simulink model "Pt_Center_Diff_CS9"  (Simulink 7.6)
settings: Solver=ode45  StartTime=0  StopTime=20  FixedStep=TSTEP  RelTol=1e-3
PreLoadFcn:
  | cd Extensions/Simulink/pt_center_diff
  | Run_ft4wd_eclass
  | lsd_parameta_eclass
  | cd ../../..
undefined symbols (not defined in the file): LOCKED_XC_DAMP, LOCKED_XC_K, LOCKED_XC_OPT, M_DIFF_XC_TABLE, R_EFF_F_XC, R_EFF_R_XC, R_GEAR_XC, R_REAR_XC
libraries: Solver_SF x1
settings Model: Creator=ywata  LastModifiedBy=hkawanishi  ExtModeTrigMode=oneshot  ExtModeArmWhenConnect=off
settings DataIOCC: LimitDataPoints=off  SaveOutput=off  SaveTime=off  SignalLoggingName=sigsOut
settings OptimizationCC: BooleanDataType=off
settings DebuggingCC: SaveWithParameterizedLinksMsg=none  SignalResolutionControl=TryResolveAllWithWarning  SolverPrmCheckMsg=none  MultiTaskDSMMsg=warning  MultiTaskCondExecSysMsg=none  FcnCallInpInsideContextMsg=Enable All
settings HardwareCC: TargetUnknown=on
settings CodeAppCC: CustomSymbolStrType=$N$R$M_T
settings GRTTargetCC: TargetFcnLib=ansi_tfl_tmw.mat  TargetFunctionLibrary=C89/C90 (ANSI)  ModelReferenceCompliant=off  MatFileLogging=off

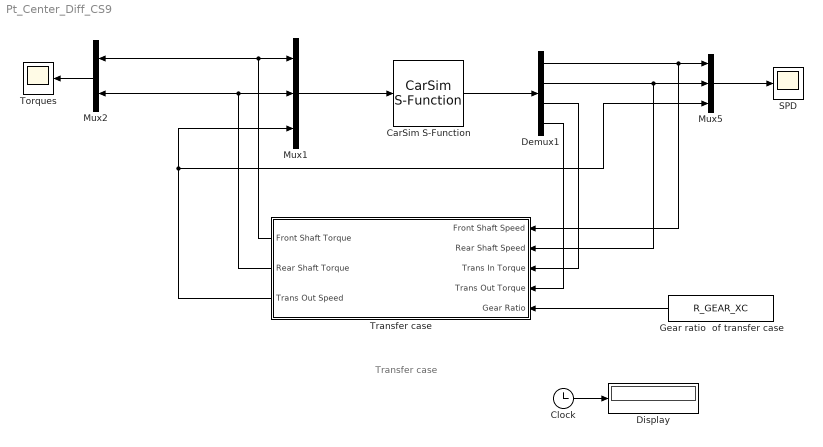
== system Pt_Center_Diff_CS9 ==
  note: Transfer case
  CarSim S-Function : Solver_SF/CarSim S-Function  Priority=1  SIMFILE=simfile.sim
  Clock : Clock
      settings: Decimation=10
  Demux1 : Demux
  Display : Display
  Gear ratio  of transfer case : Constant  Value=R_GEAR_XC
  Mux1 : Mux  Inputs=3
  Mux2 : Mux  Inputs=2
  Mux5 : Mux  Inputs=3
  SPD : Scope
      settings: YMin=-130.178  YMax=3627.22
  Torques : Scope
      settings: YMin=0  YMax=1200
  Transfer case : Subsystem
  wires:
  Mux2/1 -> Torques/1
  Mux5/1 -> SPD/1
  Gear ratio  of transfer case/1 -> Transfer case/5(Gear Ratio)
  Transfer case/3(Trans Out Speed) -> Mux1/3, Mux5/3
  Clock/1 -> Display/1
  CarSim S-Function/1 -> Demux1/1
  Mux1/1 -> CarSim S-Function/1
  Transfer case/1(Front Shaft Torque) -> Mux1/1, Mux2/1
  Transfer case/2(Rear Shaft Torque) -> Mux1/2, Mux2/2
  Demux1/1 -> Mux5/1, Transfer case/1(Front Shaft Speed)
  Demux1/2 -> Mux5/2, Transfer case/2(Rear Shaft Speed)
  Demux1/3 -> Transfer case/3(Trans In Torque)
  Demux1/4 -> Transfer case/4(Trans Out Torque)

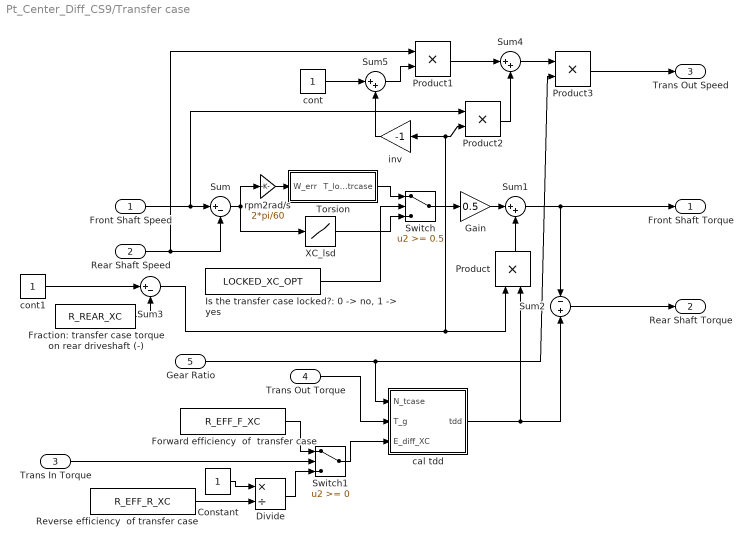
== system Pt_Center_Diff_CS9/Transfer case ==
  Front Shaft Speed : Inport
  Rear Shaft Speed : Inport  Port=2
  Trans In Torque : Inport  Port=3
  Trans Out Torque : Inport  Port=4
  Gear Ratio : Inport  Port=5
  Constant : Constant
  Divide : Product  Inputs=*/  InputSameDT=on  OutDataTypeStr=Inherit: Same as first input
  Forward efficiency  of  transfer case : Constant  Value=R_EFF_F_XC
  Fraction: transfer case torque on rear driveshaft (-) : Constant  Value=R_REAR_XC
  Gain : Gain  Gain=0.5  SaturateOnIntegerOverflow=on  OutDataTypeStr=Inherit: Same as input  ParamDataTypeStr=Inherit: Same as input
  "Is the transfer case locked?: 0 -> no, 1 -> yes" : Constant  Value=LOCKED_XC_OPT
  Product{,1..3} (4 alike) : Product  SaturateOnIntegerOverflow=on  InputSameDT=on  OutDataTypeStr=Inherit: Same as first input
  Reverse efficiency  of transfer case : Constant  Value=R_EFF_R_XC
  Sum : Sum  Inputs=|+-  SaturateOnIntegerOverflow=on  InputSameDT=on  OutDataTypeStr=Inherit: Same as first input
  Sum1 : Sum  Inputs=|++  SaturateOnIntegerOverflow=on  InputSameDT=on  OutDataTypeStr=Inherit: Same as first input
  Sum2 : Sum  Inputs=-|+  SaturateOnIntegerOverflow=on  InputSameDT=on  OutDataTypeStr=Inherit: Same as first input
  Sum3 : Sum  Inputs=|+-  SaturateOnIntegerOverflow=on  InputSameDT=on  OutDataTypeStr=Inherit: Same as first input
  Sum4 : Sum  Inputs=|++  SaturateOnIntegerOverflow=on  InputSameDT=on  OutDataTypeStr=Inherit: Same as first input
  Sum5 : Sum  Inputs=|++  SaturateOnIntegerOverflow=on  InputSameDT=on  OutDataTypeStr=Inherit: Same as first input
  Switch : Switch  Threshold=0.5  SaturateOnIntegerOverflow=on  InputSameDT=on
  Switch1 : Switch  SaturateOnIntegerOverflow=on  InputSameDT=on
  Torsion : Subsystem
  XC_lsd : Lookup  InputValues=M_DIFF_XC_TABLE(:,1)  Table=M_DIFF_XC_TABLE(:,2)  SaturateOnIntegerOverflow=on
  cal tdd : Subsystem
  cont : Constant
  cont1 : Constant
  inv : Gain  Gain=-1  SaturateOnIntegerOverflow=on  OutDataTypeStr=Inherit: Same as input  ParamDataTypeStr=Inherit: Same as input
  rpm2rad/s : Gain  Gain=2*pi/60  SaturateOnIntegerOverflow=on  OutDataTypeStr=Inherit: Same as input  ParamDataTypeStr=Inherit: Same as input
  Front Shaft Torque : Outport
  Rear Shaft Torque : Outport  Port=2
  Trans Out Speed : Outport  Port=3
  wires:
  Sum1/1 -> Sum2/1, Front Shaft Torque/1
  Sum2/1 -> Rear Shaft Torque/1
  cal tdd/1(tdd) -> Product/2, Sum2/2
  Switch1/1 -> cal tdd/3(E_diff_XC)
  Forward efficiency  of  transfer case/1 -> Switch1/1
  Trans In Torque/1 -> Switch1/2
  Trans Out Torque/1 -> cal tdd/2(T_g)
  Product/1 -> Sum1/2
  Gain/1 -> Sum1/1
  Switch/1 -> Gain/1
  "Is the transfer case locked?: 0 -> no, 1 -> yes"/1 -> Switch/2
  Sum/1 -> rpm2rad/s/1, XC_lsd/1
  Torsion/1(T_lock_trcase) -> Switch/1
  Product2/1 -> Sum4/2
  Product1/1 -> Sum4/1
  Sum4/1 -> Product3/1
  Product3/1 -> Trans Out Speed/1
  Gear Ratio/1 -> cal tdd/1(N_tcase), Product3/2
  Sum5/1 -> Product1/2
  cont/1 -> Sum5/1
  inv/1 -> Sum5/2
  Front Shaft Speed/1 -> Sum/1, Product2/1
  Rear Shaft Speed/1 -> Sum/2, Product1/1
  Fraction: transfer case torque on rear driveshaft (-)/1 -> Sum3/2
  Sum3/1 -> Product/1, Product2/2, inv/1
  cont1/1 -> Sum3/1
  Constant/1 -> Divide/1
  Reverse efficiency  of transfer case/1 -> Divide/2
  Divide/1 -> Switch1/3
  rpm2rad/s/1 -> Torsion/1(W_err)
  XC_lsd/1 -> Switch/3

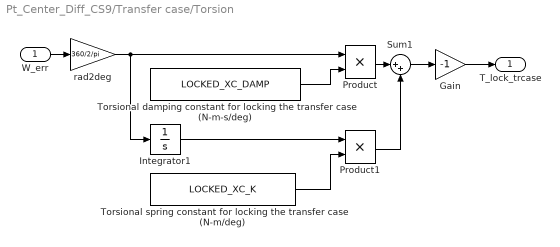
== system Pt_Center_Diff_CS9/Transfer case/Torsion ==
  W_err : Inport
  Gain : Gain  Gain=-1  SaturateOnIntegerOverflow=on  OutDataTypeStr=Inherit: Same as input  ParamDataTypeStr=Inherit: Same as input
  Integrator1 : Integrator
  Product : Product  SaturateOnIntegerOverflow=on  InputSameDT=on  OutDataTypeStr=Inherit: Same as first input
  Product1 : Product  SaturateOnIntegerOverflow=on  InputSameDT=on  OutDataTypeStr=Inherit: Same as first input
  Sum1 : Sum  Inputs=|++  SaturateOnIntegerOverflow=on  InputSameDT=on  OutDataTypeStr=Inherit: Same as first input
  Torsional damping constant for locking the transfer case (N-m-s/deg) : Constant  Value=LOCKED_XC_DAMP
  Torsional spring constant for locking the transfer case (N-m/deg) : Constant  Value=LOCKED_XC_K
  rad2deg : Gain  Gain=360/2/pi  SaturateOnIntegerOverflow=on  OutDataTypeStr=Inherit: Same as input  ParamDataTypeStr=Inherit: Same as input
  T_lock_trcase : Outport
  wires:
  Torsional spring constant for locking the transfer case (N-m/deg)/1 -> Product1/2
  Integrator1/1 -> Product1/1
  Torsional damping constant for locking the transfer case (N-m-s/deg)/1 -> Product/2
  Product/1 -> Sum1/1
  Product1/1 -> Sum1/2
  Sum1/1 -> Gain/1
  Gain/1 -> T_lock_trcase/1
  W_err/1 -> rad2deg/1
  rad2deg/1 -> Product/1, Integrator1/1

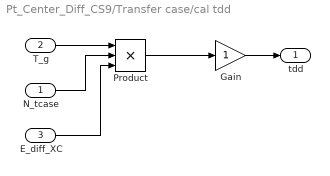
== system Pt_Center_Diff_CS9/Transfer case/cal tdd ==
  N_tcase : Inport
  T_g : Inport  Port=2
  E_diff_XC : Inport  Port=3
  Gain : Gain  SaturateOnIntegerOverflow=on  OutDataTypeStr=Inherit: Same as input  ParamDataTypeStr=Inherit: Same as input
  Product : Product  Inputs=3  SaturateOnIntegerOverflow=on  InputSameDT=on  OutDataTypeStr=Inherit: Same as first input
  tdd : Outport
  wires:
  T_g/1 -> Product/1
  N_tcase/1 -> Product/2
  E_diff_XC/1 -> Product/3
  Product/1 -> Gain/1
  Gain/1 -> tdd/1
